simulink model "motor_speed"  (R2013b)
settings: Solver=ode45  StartTime=0.0  StopTime=50  RelTol=1e-3
values from neighbouring files (symbols this model uses):
  b = I_free*K_t/nl_speed    (= 1.83906430469e-06)    [parameter_motor.m]
  J_eq = Jw    (= 8.9522375e-05)    [parameter_motor.m]
  K_b = (Vm-I_free*R)/nl_speed    (= 0.00979236958951)    [parameter_motor.m]
  K_t = T_stall/I_stall    (= 0.0070615)    [parameter_motor.m]
  L = 0.5    [parameter_motor.m]
  R = 0.001    [kalman_filter.m]    (also in parameter_motor.m = 2.4)
undefined symbols (not defined in the file or in its folder): sigbuilder_block
libraries: simulink x1
settings Model: Creator=sanjay  LastModifiedBy=sanjay

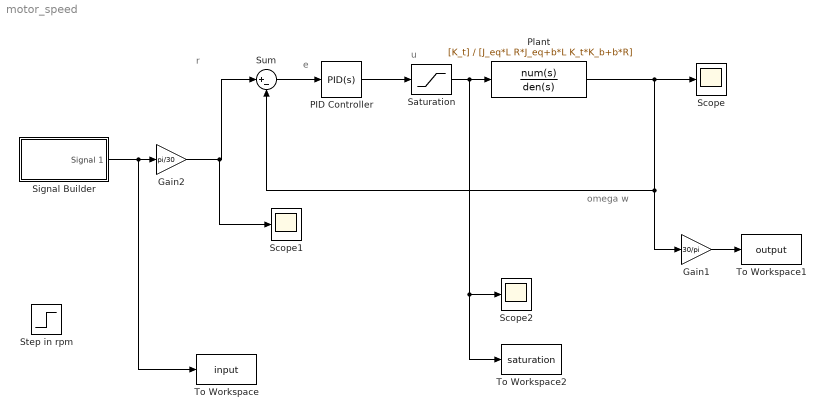
== system motor_speed ==
  note: u
  note: e
  note: omega w
  note: r
  Gain1 : Gain  Gain=30/pi
  Gain2 : Gain  Gain=pi/30
  PID Controller : simulink/Continuous/PID Controller  RequirementInfo={'other' '..\controller values.xlsx' '@Simulink_requirement_item_1' 'true' 'iter1' '' ; 'other' '..\controller values.xlsx' '@Simulink_requirement_item_1' 'true' '' '' ; 'other' '..\controller values.xlsx' '@Simulink_requirement_item_2' 'true' '' '' } %GIDa_fbdd2cd8_7785_42e6_8e75_0620455e6e7c  Controller=PID  TimeDomain=Continuous-time  SampleTime=0.000001  IntegratorMethod=Forward Euler  FilterMethod=Forward Euler  Form=Parallel  P=0.141847319632733  I=0.0533184625505999  D=0.00904700213625541  N=10.9506820386323  InitialConditionSource=internal  InitialConditionForIntegrator=0  InitialConditionForFilter=0  ExternalReset=none  LimitOutput=off  UpperSaturationLimit=inf  LowerSaturationLimit=-inf  LinearizeAsGain=on  AntiWindupMode=none  Kb=1  TrackingMode=off  Kt=1  PParamMin=[]  PParamMax=[]  IParamMin=[]  IParamMax=[]  DParamMin=[]  DParamMax=[]  NParamMin=[]  NParamMax=[]  KbParamMin=[]  KbParamMax=[]  KtParamMin=[]  KtParamMax=[]  POutMin=[]  POutMax=[]  IOutMin=[]  IOutMax=[]  DOutMin=[]  DOutMax=[]  NOutMin=[]  NOutMax=[]  KbOutMin=[]  KbOutMax=[]  KtOutMin=[]  KtOutMax=[]  IntegratorOutMin=[]  IntegratorOutMax=[]  FilterOutMin=[]  FilterOutMax=[]  SumOutMin=[]  SumOutMax=[]  SumI1OutMin=[]  SumI1OutMax=[]  SumI2OutMin=[]  SumI2OutMax=[]  SumI3OutMin=[]  SumI3OutMax=[]  SumDOutMin=[]  SumDOutMax=[]  SaturationOutMin=[]  SaturationOutMax=[]  IntegratorContinuousStateAttributes=''  IntegratorStateMustResolveToSignalObject=off  IntegratorRTWStateStorageClass=Auto  FilterContinuousStateAttributes=''  FilterStateMustResolveToSignalObject=off  FilterRTWStateStorageClass=Auto
  Plant : TransferFcn  Numerator=[K_t]  Denominator=[J_eq*L R*J_eq+b*L K_t*K_b+b*R]
  Saturation : Saturate  UpperLimit=9  LowerLimit=-9
  Scope : Scope
      settings: TimeRange=1000  YMin=0  YMax=1200
  Scope1 : Scope
      settings: TimeRange=1000  YMin=0  YMax=1200
  Scope2 : Scope
      settings: TimeRange=1000  YMin=0  YMax=1200  SaveName=ScopeData2
  Signal Builder : Subsystem  Tag=STV Subsys  LoadFcn=sigbuilder_block('load');  StartFcn=sigbuilder_block('start');  StopFcn=sigbuilder_block('stop');  ClipboardFcn=sigbuilder_block('clipboard');  mask(Sigbuilder block){}
      mask help: Simulink:masks:SigbuilderBlock_MD
      mask init:
      | if ~strcmp(get_param(bdroot(gcbh),'SimulationStatus'),'stopped') tuvar = sigbuilder_block('maskInit'); end
      settings: CopyFcn=sigbuilder_block('copy');  DeleteFcn=sigbuilder_block('delete');  ModelCloseFcn=sigbuilder_block('modelClose');  PreSaveFcn=sigbuilder_block('preSave');  PauseFcn=sigbuilder_block('pause');  ContinueFcn=sigbuilder_block('continue');  NameChangeFcn=sigbuilder_block('namechange');  OpenFcn=sigbuilder_block('open',[437.25 117.75 550.5 394.5 ]);  CloseFcn=sigbuilder_block('close');
      mask Display: plot(0, 0, 100, 100,[2, 2, 32, 32, 2], [68, 8, 8, 68, 68],[32, 2], [38, 38], [32, 19, 2],[53, 60, 44], [32, 17, 17, 2],[16, 16, 31, 31]);txt = getActiveGroup(gcbh);text(2, 100, txt,'verticalAlignment', 'top');
  Step in rpm : Step  After=20*pi/3  SampleTime=0
  Sum : Sum  Inputs=|+-
  To Workspace : ToWorkspace  VariableName=input  SampleTime=-1  SaveFormat=Timeseries
  To Workspace1 : ToWorkspace  VariableName=output  SampleTime=-1  SaveFormat=Timeseries
  To Workspace2 : ToWorkspace  VariableName=saturation  SampleTime=-1  SaveFormat=Timeseries
  wires:
  PID Controller/1 -> Saturation/1
  Saturation/1 -> Scope2/1, To Workspace2/1, Plant/1
  Plant/1 -> Scope/1, Sum/2, Gain1/1
  Sum/1 -> PID Controller/1
  Gain1/1 -> To Workspace1/1
  Gain2/1 -> Scope1/1, Sum/1
  Signal Builder/1(Signal 1) -> To Workspace/1, Gain2/1

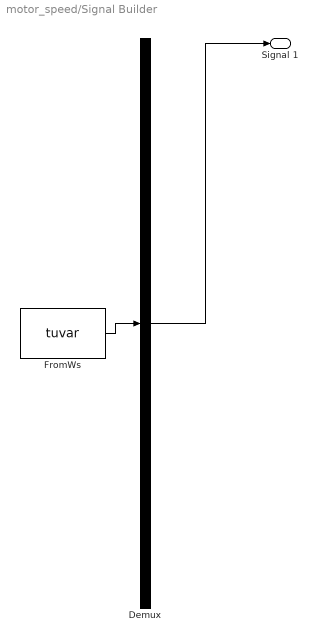
== system motor_speed/Signal Builder ==
  Demux : Demux  Tag=STV Demux  Outputs=1
  FromWs : FromWorkspace  Tag=STV FromWs  VariableName=tuvar  SampleTime=0
      SigBuilderData=|
      | common.afterFinalStr = 'Extrapolate'
      | common.sampleTime = 0
      | dataSet.timeRange = [0 20]
      | dataSet.name = 'Group 1'
      | sbobj.Groups.Name = 'Group 1'
      | sbobj.Groups.Signals.Name = 'Signal 1'
      | sbobj.Groups.Signals.XData = [0 2 4 6 8 10 20]
      | sbobj.Groups.Signals.YData = [0 21 100 79.5 23.5 0 0]
      | sbobj.Groups.TimeRange = [0 20]
  Signal 1 : Outport  Tag=STV Outport
  wires:
  Demux/1 -> Signal 1/1
  FromWs/1 -> Demux/1
